simulink model "MILSILmultistop"  (R2023a)
settings: Solver=FixedStepDiscrete  StartTime=0.0  StopTime=10.0  RelTol=1e-3
values from neighbouring files (symbols this model uses):
  goal = [-273.049453636 -165.667646685 232.685507806]    [plannerworkspace.mat]
  newedgeTable = [1 2 3 4 5 6 7 8 9 10 11 12 ... (29452 elements, 14726x2)]    [plannerworkspace.mat]
  newnodeTable = [-55.6615304834 -55.7711747144 -55.906310259 -56.0027958259 -56.044091125 -56.1593867623 -56.1684563435 -56.1721227456 -56.2079408409 -56.2275338603 -56.2371618722 -56.2272355877 ... (43533 elements, 14511x3)]    [plannerworkspace.mat]
  start = [49.3593481885 176.940631309 239.210089237]    [plannerworkspace.mat]
settings Model: Creator=greys  LastModifiedBy=greys
settings OptimizationCC: DefaultParameterBehavior=Inlined  UseDivisionForNetSlopeComputation=on  GainParamInheritBuiltInType=on  UseFloatMulNetSlope=on  OptimizeBlockIOStorage=off
settings HardwareCC: TargetBitPerPointer=64  TargetBitPerSizeT=64  TargetBitPerPtrDiffT=64  TargetLongLongMode=on  TargetIntDivRoundTo=Zero  TargetEndianess=LittleEndian  TargetWordSize=64  TargetHWDeviceType=MATLAB Host  ProdEqTarget=off
settings RTWCC: GenCodeOnly=on  GenerateReport=on  BuildConfiguration=Debug  LaunchReport=on  CodeExecutionProfiling=on  CodeProfilingSaveOptions=AllData
settings CodeAppCC: ForceParamTrailComments=on  MATLABSourceComments=on

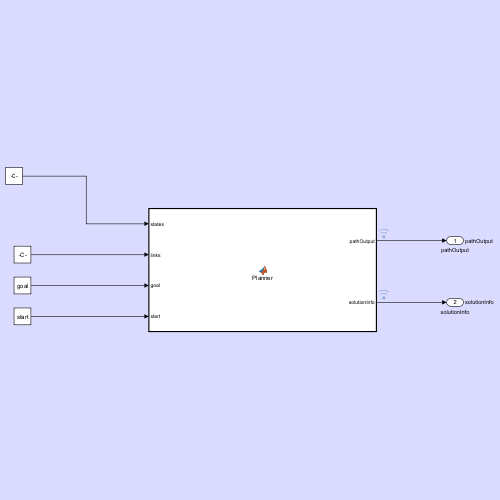
[thumbnail: Simulink's stored preview of the top-level diagram]
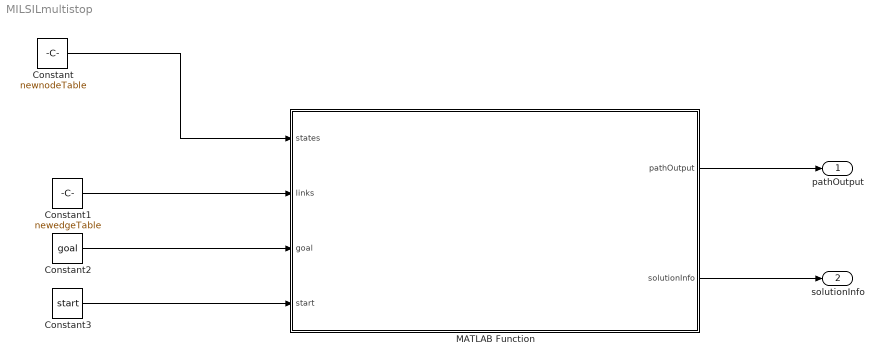
== system MILSILmultistop ==
  Constant : Constant  Value=newnodeTable  VectorParams1D=off  SampleTime=-1
  Constant1 : Constant  Value=newedgeTable  VectorParams1D=off
  Constant2 : Constant  Value=goal  VectorParams1D=off
  Constant3 : Constant  Value=start  VectorParams1D=off
  MATLAB Function : MATLAB Function  TreatAsAtomicUnit=on
  pathOutput : Outport  SignalName=pathOutput  OutMin=0  OutMax=10  PortDimensions=[1000 3]  SampleTime=1
  solutionInfo : Outport  Port=2  SignalName=solutionInfo  OutMin=[0]  OutMax=[1]
  wires:
  Constant3/1 -> MATLAB Function/4(start)
  Constant2/1 -> MATLAB Function/3(goal)
  Constant1/1 -> MATLAB Function/2(links)
  MATLAB Function/2(solutionInfo) -> solutionInfo/1
  MATLAB Function/1(pathOutput) -> pathOutput/1
  Constant/1 -> MATLAB Function/1(states)

== matlab function MILSILmultistop/MATLAB Function ==
  data: states input; links input; goal input; start input size=3; pathOutput output double size=[1000 3]; solutionInfo output boolean size=1 [0..1]
function [pathOutput,solutionInfo] = Planner(states,links,goal,start)

%PLANNER Summary of this function goes here
%   Detailed explanation goes here
start=transpose(start);
graphObj = navGraph(states,links);
planner = plannerAStar(graphObj);
pathOutput=zeros(1000,3);
[pathOutput1,solutionInfo1] = plan(planner,start,goal);
if size(pathOutput1)~=0
    pathOutput([1,size(pathOutput1,1)],:)=pathOutput1([1,size(pathOutput1,1)],:);
end
solutionInfo=solutionInfo1.IsPathFound;
